simulink model "Projekt_model"  (R2012b)
settings: Solver=ode45  StartTime=0.0  StopTime=10.0  RelTol=1e-3
settings Model: Creator=Vallen  LastModifiedBy=Vallen

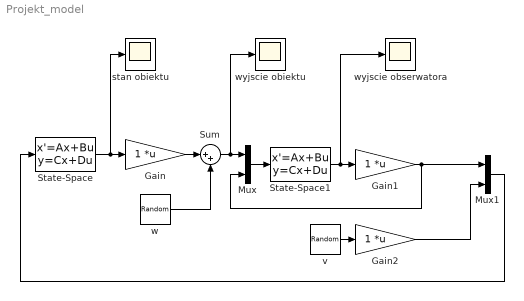
== system Projekt_model ==
  Gain : Gain  Multiplication=Matrix(K*u) (u vector)
  Gain1 : Gain  Multiplication=Matrix(K*u) (u vector)
  Gain2 : Gain  Multiplication=Matrix(K*u) (u vector)
  Mux : Mux  Inputs=2
  Mux1 : Mux  Inputs=2
  State-Space : StateSpace
  State-Space1 : StateSpace
  Sum : Sum  Inputs=|++
  stan obiektu : Scope
  v : RandomNumber  SampleTime=0.1
  w : RandomNumber  SampleTime=0.1
  wyjscie obiektu : Scope
  wyjscie obserwatora : Scope
      settings: SaveName=ScopeData2
  wires:
  State-Space/1 -> stan obiektu/1, Gain/1
  Gain/1 -> Sum/1
  w/1 -> Sum/2
  Sum/1 -> wyjscie obiektu/1, Mux/1
  Mux/1 -> State-Space1/1
  State-Space1/1 -> wyjscie obserwatora/1, Gain1/1
  Gain1/1 -> Mux1/1, Mux/2
  v/1 -> Gain2/1
  Gain2/1 -> Mux1/2
  Mux1/1 -> State-Space/1
